simulink model "sim_model"  (R2021b)
settings: Solver=ode1  StartTime=0.0  StopTime=6e3  FixedStep=1  RelTol=1e-3
values from neighbouring files (symbols this model uses):
  Cd = 1    [MainNMPC.m]    (also in Parameters.m = 2.2; matlab.mat)
  coeffT = Tmax/g0/Isp    (= 0.00101971621298)    [MainNMPC.m]    (also in Parameters.m; matlab.mat)
  endOrbit_v = [orb_end.a orb_end.e orb_end.i orb_end.OM orb_end.om traj_state(6,end)]'    [MainNMPC.m]    (also in matlab.mat = [10000 0.2 0.785398163397 0 1.0471975512 449.308981824])
  initOrbit_v = [orb_in.a orb_in.e orb_in.i orb_in.OM orb_in.om traj_state(6,1)]'    [MainNMPC.m]    (also in matlab.mat = [8000 0 0.785398163397 0 0 2.52094315108])
  M = 20    [MainNMPC.m]    (also in Parameters.m; matlab.mat = 100)
  m0 = 1000    [MainNMPC.m]    (also in Parameters.m; matlab.mat)
  mu = 398600    [MainNMPC.m]    (also in Parameters.m; matlab.mat; mySQP.m = zeros(options.nitermax+1, q)'; mu(:,1) = zeros(q,1))
  S = 1    [MainNMPC.m]    (also in Parameters.m = 5; matlab.mat)
  traj_angle = makima(topt,alphaCell{8}(lu+2:end)',t)    [MainNMPC.m]    (also in matlab.mat = [1.81279639193 1.76244926401 1.72305689141 1.69378795925 1.6)
  traj_csi = makima(topt,alphaCell{8}(2:lu+1)',t)    [MainNMPC.m]    (also in matlab.mat = [0.0167214416109 0.0144924734441 0.0121999637993 0.009914142)
  traj_state = alphaCell{14}    [MainNMPC.m]    (also in matlab.mat = [8000 0 0 0.414213562373 0 2.52094315108 7999.99091681 2.261)
  Ts = 100    [MainNMPC.m]    (also in MoonModel.m; Parameters.m; matlab.mat; moonDisturbance.m)
  x_par = fminsearch(funX,initX)    [MoonModel.m]    (also in matlab.mat = [-21743.4033853 2.01148903137 2.66443158727e-06 380984.58833; moonModelParams.mat = [-21745.1690869 2.01149208089 2358171.82299 380982.473681])
  y_par = fminsearch(funY,initY)    [MoonModel.m]    (also in matlab.mat = [25727.2862258 0.485798378776 2.66290385777e-06 339518.69935; moonModelParams.mat = [25725.8292628 0.485807216446 2359526.4503 339520.022873])
  z_par = fminsearch(funZ,initZ)    [MoonModel.m]    (also in matlab.mat = [14641.8884076 0.343953021327 2.66655675453e-06 176611.97281; moonModelParams.mat = [14641.6479642 0.34394662724 2356290.20223 176611.681536])
libraries: simulink x1
settings Model: Creator=matteodepaola  LastModifiedBy=matteodepaola

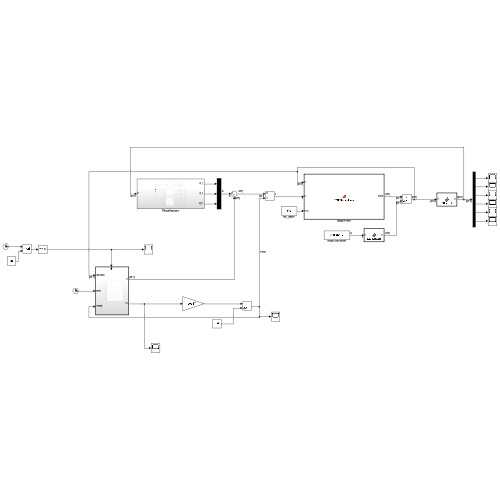
[thumbnail: Simulink's stored preview of the top-level diagram]
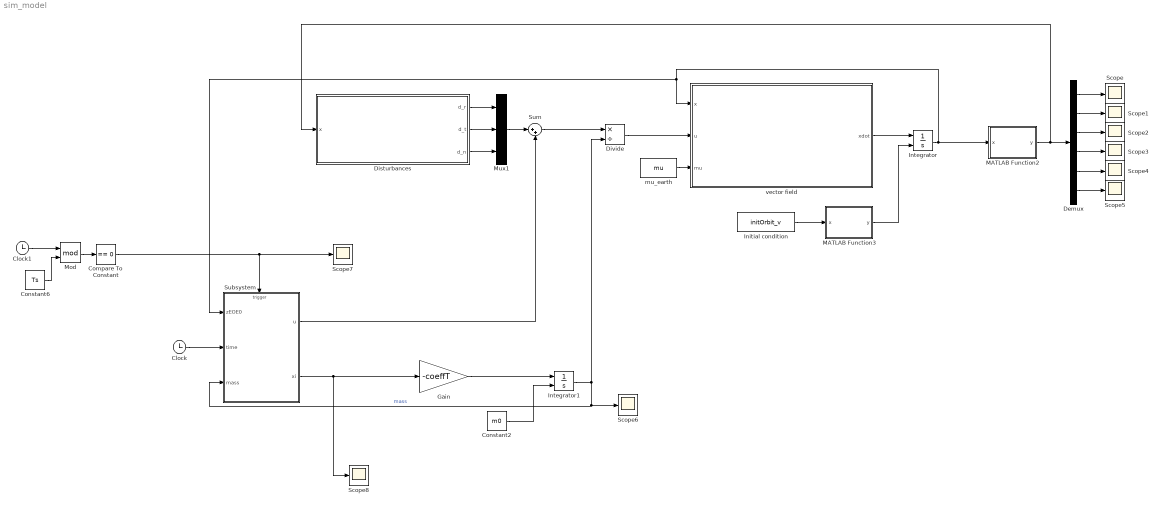
== system sim_model ==
  Clock : Clock
  Clock1 : Clock
  Compare To Constant : simulink/Logic and Bit Operations/Compare To Constant  relop===  const=0  OutDataTypeStr=boolean
  Constant2 : Constant  Value=m0
  Constant6 : Constant  Value=Ts
  Demux : Demux  Outputs=6
  Disturbances : Subsystem
  Divide : Product  Inputs=*/
  Gain : Gain  Gain=-coeffT
  Initial condition : Constant  Value=initOrbit_v
  Integrator : Integrator  InitialConditionSource=external
  Integrator1 : Integrator  InitialConditionSource=external  InitialCondition=1500
  MATLAB Function2 : MATLAB Function  TreatAsAtomicUnit=on
  MATLAB Function3 : MATLAB Function  TreatAsAtomicUnit=on
  Mod : Math  Operator=mod  SaturateOnIntegerOverflow=on
  Mux1 : Mux  Inputs=3
  Scope{,1..8} (9 alike) : Scope
  Subsystem : Subsystem
  Sum : Sum  Inputs=|++
  mu_earth : Constant  Value=mu
  vector field : MATLAB Function  TreatAsAtomicUnit=on
  wires:
  vector field/1(xdot) -> Integrator/1
  mu_earth/1 -> vector field/3(mu)
  Disturbances/1(d_r) -> Mux1/1
  Disturbances/2(d_t) -> Mux1/2
  Disturbances/3(d_n) -> Mux1/3
  Integrator1/1 -> Scope6/1, Subsystem/3(mass), Divide/2  "mass"
  Mux1/1 -> Sum/1
  Integrator/1 -> Subsystem/1(zEOE0), vector field/1(x), MATLAB Function2/1(x)
  MATLAB Function2/1(y) -> Demux/1, Disturbances/1(x)
  Initial condition/1 -> MATLAB Function3/1(x)
  MATLAB Function3/1(y) -> Integrator/2
  Gain/1 -> Integrator1/1
  Sum/1 -> Divide/1
  Constant2/1 -> Integrator1/2
  Divide/1 -> vector field/2(u)
  Demux/1 -> Scope/1
  Demux/2 -> Scope1/1
  Demux/3 -> Scope2/1
  Demux/4 -> Scope3/1
  Demux/5 -> Scope4/1
  Demux/6 -> Scope5/1
  Clock1/1 -> Mod/1
  Constant6/1 -> Mod/2
  Mod/1 -> Compare To Constant/1
  Compare To Constant/1 -> Scope7/1, Subsystem/Trigger
  Clock/1 -> Subsystem/2(time)
  Subsystem/1(u) -> Sum/2
  Subsystem/2(xi) -> Scope8/1, Gain/1

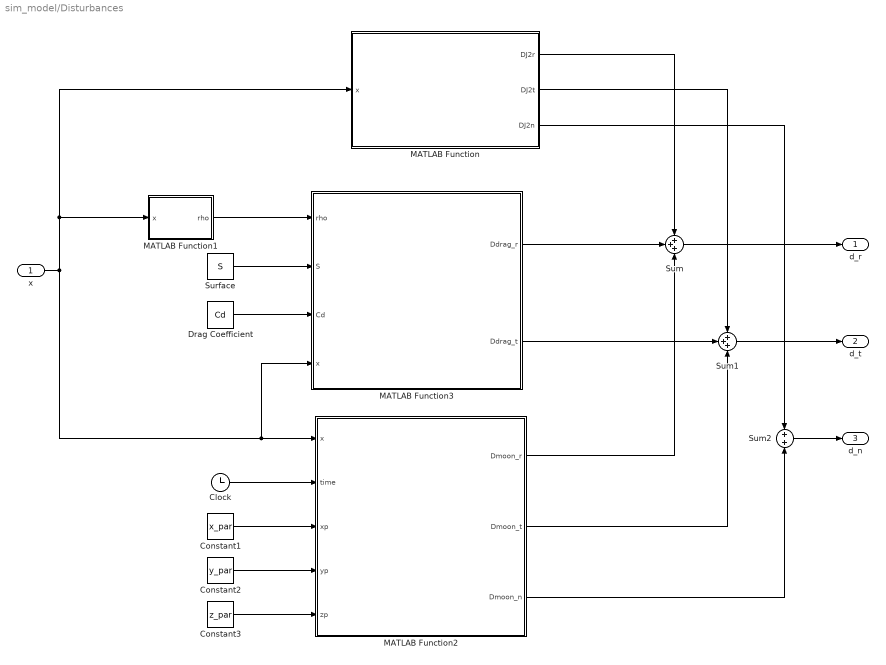
== system sim_model/Disturbances ==
  x : Inport
  Clock : Clock
  Constant1 : Constant  Value=x_par
  Constant2 : Constant  Value=y_par
  Constant3 : Constant  Value=z_par
  Drag Coefficient : Constant  Value=Cd
  MATLAB Function : MATLAB Function  TreatAsAtomicUnit=on
  MATLAB Function1 : MATLAB Function  TreatAsAtomicUnit=on
  MATLAB Function2 : MATLAB Function  TreatAsAtomicUnit=on
  MATLAB Function3 : MATLAB Function  TreatAsAtomicUnit=on
  Sum : Sum  Inputs=+++
  Sum1 : Sum  Inputs=+++
  Sum2 : Sum  Inputs=+|+
  Surface : Constant  Value=S
  d_r : Outport
  d_t : Outport  Port=2
  d_n : Outport  Port=3
  wires:
  MATLAB Function/3(DJ2n) -> Sum2/1
  x/1 -> MATLAB Function/1(x), MATLAB Function1/1(x), MATLAB Function3/4(x), MATLAB Function2/1(x)
  MATLAB Function/1(DJ2r) -> Sum/1
  MATLAB Function1/1(rho) -> MATLAB Function3/1(rho)
  Clock/1 -> MATLAB Function2/2(time)
  Drag Coefficient/1 -> MATLAB Function3/3(Cd)
  MATLAB Function3/1(Ddrag_r) -> Sum/2
  Surface/1 -> MATLAB Function3/2(S)
  MATLAB Function2/1(Dmoon_r) -> Sum/3
  MATLAB Function/2(DJ2t) -> Sum1/1
  MATLAB Function3/2(Ddrag_t) -> Sum1/2
  MATLAB Function2/2(Dmoon_t) -> Sum1/3
  MATLAB Function2/3(Dmoon_n) -> Sum2/2
  Sum/1 -> d_r/1
  Sum1/1 -> d_t/1
  Sum2/1 -> d_n/1
  Constant1/1 -> MATLAB Function2/3(xp)
  Constant2/1 -> MATLAB Function2/4(yp)
  Constant3/1 -> MATLAB Function2/5(zp)

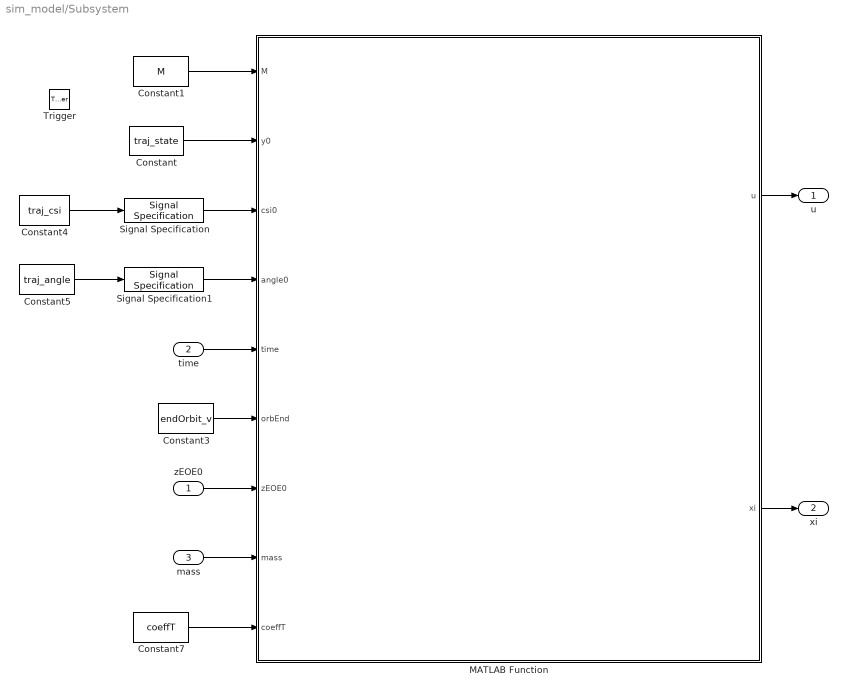
== system sim_model/Subsystem ==
  zEOE0 : Inport
  time : Inport  Port=2
  mass : Inport  Port=3
  Trigger : TriggerPort  VariantControl=(inherit)  PortDimensions=1
  Constant : Constant  Value=traj_state
  Constant1 : Constant  Value=M
  Constant3 : Constant  Value=endOrbit_v
  Constant4 : Constant  Value=traj_csi
  Constant5 : Constant  Value=traj_angle
  Constant7 : Constant  Value=coeffT
  MATLAB Function : MATLAB Function  TreatAsAtomicUnit=on
  Signal Specification : SignalSpecification  Dimensions=[1,6001]
  Signal Specification1 : SignalSpecification  Dimensions=[1,6001]
  u : Outport
  xi : Outport  Port=2
  wires:
  Constant3/1 -> MATLAB Function/6(orbEnd)
  Constant5/1 -> Signal Specification1/1
  Constant1/1 -> MATLAB Function/1(M)
  MATLAB Function/2(xi) -> xi/1
  zEOE0/1 -> MATLAB Function/7(zEOE0)
  Constant/1 -> MATLAB Function/2(y0)
  mass/1 -> MATLAB Function/8(mass)
  Constant4/1 -> Signal Specification/1
  Constant7/1 -> MATLAB Function/9(coeffT)
  time/1 -> MATLAB Function/5(time)
  MATLAB Function/1(u) -> u/1
  Signal Specification/1 -> MATLAB Function/3(csi0)
  Signal Specification1/1 -> MATLAB Function/4(angle0)

== matlab function sim_model/Disturbances/MATLAB Function1 ==
  data: x input; rho output
function rho = rho_selection(x)
a = x(1);
e = x(2);
theta = x(6);

% [km kg/m^3 km] % check Bernelli slides for references
rho_table = [0 1.225 7.249 ;
    25 3.899e-2 6.349 ;
    30 1.774e-2 6.682 ;
    40 3.972e-3 7.554 ;
    50 1.057e-3 8.382 ;
    60 3.206e-4 7.714 ;
    70 8.770e-5 6.549 ;
    80 1.905e-5 5.779 ;
    90 3.396e-6 5.382 ;
    100 5.297e-7 5.877 ;
    110 9.661e-8 7.263 ;
    120 2.438e-8 9.473 ;
    130 8.484e-9 12.636 ;
    140 3.845e-9 16.149 ;
    150 2.070e-9 22.523 ;
    180 5.464e-10 29.740 ;
    200 2.789e-10 37.105 ;
    250 7.248e-11 45.548 ;
    300 2.418e-11 53.628 ;
    350 9.158e-12 53.298 ;
    400 3.725e-12 58.515 ;
    450 1.585e-12 60.828 ;
    500 6.967e-13 63.822 ;
    600 1.454e-13 71.835 ;
    700 3.614e-14 88.667 ;
    800 1.170e-14 124.64 ;
    900 5.245e-15 181.05 ;
    1000 3.019e-15 268.00];


p = a*(1-e^2); % semilatum rectum [km]
r = p/(1+e*cos(theta)); % distance from focus in km
earth_radius = 6.3781e+3; %[km] %correction, before it was e+6
h = r - earth_radius; %[km]
% R = sqrt(r^2+(e*a)^2+2*r*e*a*cos(theta)) % distance from earth

%selection of rho_
select = 0;

for ind = 2:28
    if h < rho_table(ind,1)
        select = ind - 1;
        break
    end
end

if select == 0
    select = 28;
end

h_0     =   rho_table(select, 1);
rho_0   =   rho_table(select, 2);
H       =   rho_table(select, 3);
rho = rho_0*exp(-(h-h_0)/H);

== matlab function sim_model/Disturbances/MATLAB Function ==
  data: x input; DJ2r output; DJ2t output; DJ2n output
function[DJ2r, DJ2t, DJ2n] = earthNonSphericity(x)

J2 = 0.001082;  % geopotential coefficient of earth's oblateness
mu_earth = 398600;    % [km^3*s^-3] standard gravitational parameter of earh (mu = G*M)
Re = 6371;      % [km] earth equatorial radius

a = x(1);
e = x(2);
i = x(3);
Omega = x(4);
w = x(5);
theta = x(6);

h = cos(Omega)*tan(i/2);
k = sin(Omega)*tan(i/2);
L = Omega+w+theta;

[rr,~] = paraorb2rv(a,e,i,Omega,w,theta,mu_earth);

r = sqrt(rr(1)^2+rr(2)^2+rr(3)^2);

DJ2r = -(3*mu_earth*J2*Re^2)/(2*r^4)*(1-12*(h*sin(L)-k*cos(L)^2)/(1+h^2+k^2)^2);
DJ2t = -(12*mu_earth*J2*Re^2)/(r^4)*(h*sin(L)-k*cos(L))*(h*cos(L)+k*sin(L))/(1+h^2+k^2)^2;
DJ2n = -(6*mu_earth*J2*Re^2)/(r^4)*(1-h^2-k^2)*(h*sin(L)-k*cos(L))/(1+h^2+k^2)^2;

== matlab function sim_model/Disturbances/MATLAB Function2 ==
  data: x input; time input; xp input; Dmoon_r output; Dmoon_t output; Dmoon_n output; yp input; zp input
function [Dmoon_r, Dmoon_t, Dmoon_n]  = moonDisturbance(x, time, xp, yp, zp)

a = x(1);
e = x(2);
i = x(3);
Omega = x(4);
w = x(5);
theta = x(6);

mu_earth = 398600;
Ts = 100;
[r,v] = paraorb2rv(a,e,i,Omega,w,theta,mu_earth);
r = r';
v = v';

k = floor(time/Ts)*Ts;

x_m = xp(1)+xp(4)*sin(xp(3)*k+xp(2));
y_m = yp(1)+yp(4)*sin(yp(3)*k+yp(2));
z_m = zp(1)+zp(4)*sin(zp(3)*k+zp(2));
s = [x_m; y_m; z_m];

% r position vector of the spacecraft
% time is the value representing the Julian day in TDT scale

mu_moon = 490487;               % moon standard gravitational coefficient

d = r-s;                            % vector from moon to spacecraft
d_mod = sqrt(d(1)^2+d(2)^2+d(3)^2); % modulus of d
q = r'*(r-2*s)/(s'*s);
F = @(q) q*(3+3*q+q^2)/(1+(1+q)^(3/2));

t = -mu_moon/d_mod^3*(r+F(q)*s);

ir = r/norm(r);
in = cross(r,v)/norm(cross(r,v));
it = cross(in,ir);

Q = [ir it in];

a_tb = Q*t;

Dmoon_r = a_tb(1);
Dmoon_t = a_tb(2);
Dmoon_n = a_tb(3);

== matlab function sim_model/Disturbances/MATLAB Function3 ==
  data: rho input; Ddrag_r output; S input; Cd input; x input; Ddrag_t output
function [Ddrag_r, Ddrag_t] = drag(rho,S,Cd,x)

a = x(1);
e = x(2);
i = x(3);
Omega = x(4);
w = x(5);
theta = x(6);

mu_earth = 398600;
[~,vv] = paraorb2rv(a,e,i,Omega,w,theta,mu_earth);

p = a*(1-e^2);
f = e*cos(w+Omega);
g = e*sin(w+Omega);
% h = cos(Omega)*tan(i/2);
% k = sin(Omega)*tan(i/2);
L = Omega+w+theta;


v_mod = sqrt(vv(1)^2+vv(2)^2+vv(3)^2);
v_r   = sqrt(mu_earth/p)*(f*sin(L)-g*cos(L));
v_t   = sqrt(mu_earth/p)*(1+f*cos(L)+g*sin(L));

Ddrag_r = -1/2*rho*S*Cd*v_mod*v_r;
Ddrag_t = -1/2*rho*S*Cd*v_mod*v_t;
end

== matlab function sim_model/vector field ==
  data: x input; u input; xdot output; mu input
function xdot = EOEDerivatives(x, u, mu)

% Equinoctial Orbital Elements
p = x(1);
if p < 0
    p = -p;
%     warning('p became negative. Switched to absolute value for calculations');
end
f = x(2);
g = x(3);
h = x(4);
k = x(5);
L = x(6);

% Accelerations
ar = u(1);
at = u(2);
an = u(3);

% Definition of useful values
w = 1 + f*cos(L)+g*sin(L);
% r = p/w;
s2 = 1+h^2+k^2;
% alpha2 = h^2-k^2;
p_mu05 = sqrt(p/mu);

% State Derivative Calculation
pdot = 2*p/w*p_mu05*at;
fdot = p_mu05*(ar*sin(L) + ((w+1)*cos(L)+f)*at/w - (h*sin(L)-k*cos(L))*g*an/w);
gdot = p_mu05*(-ar*cos(L) + ((w+1)*sin(L)+g)*at/w + (h*sin(L)-k*cos(L))*g*an/w);
hdot = p_mu05*s2*an/2/w*cos(L);
kdot = p_mu05*s2*an/2/w*sin(L);
Ldot = sqrt(mu*p)*(w/p)^2+p_mu05/w*(h*sin(L)-k*cos(L))*an;

xdot = [pdot fdot gdot hdot kdot Ldot]';

== matlab function sim_model/MATLAB Function2 ==
  data: x input; y output
function y  = EOE2COE(x)

%EOE2COE  Function to convert Equinoctial Orbital Elements to Classical 
%   Orbital Elements.
%   COE = EOE2COE(EOE) receives as input a vector of the 6 equinoctial OE and
%   gives as output a column vector of the 6 classical OE.
%   In particular, the input vector must be of the form EOE = [p f g h k L],
%   where p is the semilatus rectum and L is the true longitude
%   The output vector is in the form COE = [a e i om OM theta]', where
%       a: semimajor axis
%       e: eccentricity
%       i: inclination
%       om: argument of periapsis
%       OM: longitude of the ascending node
%       theta: true anomaly

p = x(1);
f = x(2);
g = x(3);
h = x(4);
k = x(5);
L = x(6);

a = p/(1-f^2-g^2);
e = sqrt(f^2+g^2);
i = atan2(2*sqrt(h^2+k^2), 1-h^2-k^2);
OM = atan2(k,h);
om = atan2(g*h-f*k, f*h+g*k);
theta = L-OM-om;

y = [a e i OM om theta]';

% u = om+theta Argument of latitude

== matlab function sim_model/MATLAB Function3 ==
  data: x input; y output
function y  = COE2EOE(x)

%COE2EOE  Function to convert Classical Orbital Elements to Equinoctial 
%   Orbital Elements.
%   EOE = COE2EOE(COE) receives as input a vector of the 6 classical OE and
%   gives as output a column vector of the 6 equinoctial OE.
%   In particular, the input vector must be of the form 
%   COE = [a e i om OM theta], where
%       a: semimajor axis
%       e: eccentricity
%       i: inclination
%       om: argument of periapsis
%       OM: longitude of the ascending node
%       theta: true anomaly
%   The output vector is in the form EOE = [p f g h k L], where p is the 
%   semilatus rectum and L is the true longitude

if isa(x, 'double')

    a = x(1);
    e = x(2);
    i = x(3);
    OM = x(4);
    om = x(5);
    theta = x(6);

elseif isa(x, 'struct')

    a = x.a;
    e = x.e;
    i = x.i;
    om = x.om;
    OM = x.OM;
    theta = x.theta;

end  

p = a*(1-e^2);
f = e*cos(om+OM);
g = e*sin(om+OM);
h = cos(OM)*tan(i/2);
k = sin(OM)*tan(i/2);
L = OM+om+theta;

y = [p f g h k L]';

== matlab function sim_model/Subsystem/MATLAB Function ==
  data: M input; u output; y0 input; csi0 input; angle0 input; time input; orbEnd input; zEOE0 input; mass input; coeffT input; xi output
function [u, xi] = NMPC(M, y0, csi0, angle0, time, orbEnd, zEOE0, mass, coeffT)

% M         Prediction horizon
% y0        Reference trajectory
% csi0      Reference fuel consumption
% angle0    Reference thruster angle
% time      Clock time
% orbEnd    Target orbit
% zEOE0     Current state in Equinoctial
% mass      Current mass
% coeffT    Maximum fuel consumption

% preinitialization
u = zeros(3,1);
xi = 0;

% trajectory generation

% trajectory initialization
Tmax = 10;
Ts = 100;    % Sampling time 
yRef = zeros(6,M);
csiRef = zeros(1,M);
angleRef = zeros(1,M);
k = floor(time/Ts); % elapsed time instants
t = length(y0)-k; % remaining points of the trajectory
d = y0(end,end)-y0(end,end-1); % last L difference

if t >= M
    yRef = y0(:,k+1:k+M);
    angleRef = angle0(k+1:k+M);
    csiRef = csi0(k+1:k+M);

elseif t < M && t > 0
    yRef(:,1:t) = y0(:,k+1:k+t);
    csiRef(1,1:t) = csi0(1,k+1:k+t);
    angleRef(1,1:t) = angle0(1,k+1:k+t);

    yRef(1:5,t+1:M) = y0(1:5,end)*ones(1,M-t);
    yRef(6,t+1:M) = y0(end,end)+d*(1:M-t);
    csiRef(1,t+1:M) = zeros(1,M-t);
    angleRef(1,t+1:M) = zeros(1,M-t);
else
    csiRef = zeros(1,M);
    angleRef = zeros(1,M);
    yRef(1:5,:) = orbEnd(1:5)*ones(1,M);
    yRef(6,:) = y0(end,end)+d*((1:M)-t);
end

% NMPC


Q = eye(6);
R = 1;

x0 = zeros(3*M,1);
x0(1:M,1) = csiRef;
x0(M+1:2*M,1) = angleRef;


coder.extrinsic("opt_problem");
xopt = opt_problem(x0,M,Ts,zEOE0,yRef,Q,R,coeffT,mass,Tmax);

xi = xopt(1);
if xi > 1
    xi = 1;
elseif xi < 0
    xi = 0;
end
u = xi*[sin(xopt(M+1,1))*cos(xopt(2*M+1,1)) cos(xopt(M+1,1))*cos(xopt(2*M+1,1)) sin(xopt(2*M+1,1))]'*Tmax/mass/1e3;
end
